simulink model "power_2rectifiers"  (Simulink 6.0)
settings: Solver=ode23tb  SolverMode=SingleTasking  StartTime=0.0  StopTime=0.1  RelTol=1e-3
libraries: powerlib x25
settings Model: Creator=sybille  LastModifiedBy=batserve  ExtModeTrigMode=oneshot  ExtModeArmWhenConnect=off  ExtModeAutoUpdateStatusClock=off
settings DataIOCC: LimitDataPoints=off  SignalLoggingName=sigsOut
settings OptimizationCC: BlockReduction=off  BooleanDataType=off
settings DebuggingCC: CheckExecutionContextPreStartOutputMsg=on  CheckExecutionContextRuntimeOutputMsg=on  SolverPrmCheckMsg=none
settings HardwareCC: TargetUnknown=on

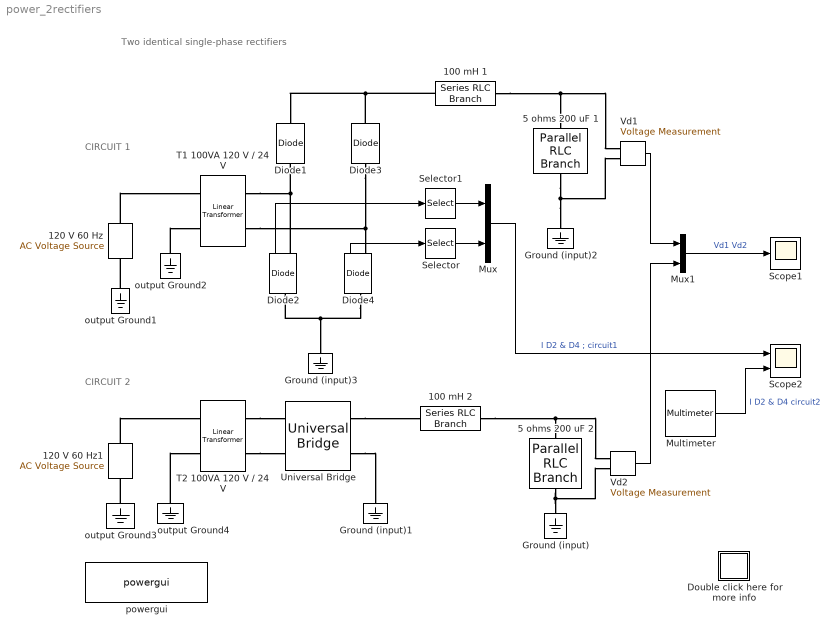
== system power_2rectifiers ==
  note: CIRCUIT 1
  note: CIRCUIT 2
  note: Two identical single-phase rectifiers
  100 mH 1 : powerlib/Elements/Series RLC Branch  PhysicalDomain=powersysdomain  SubClassName=unknown  LeftPortType=p1  RightPortType=p1  LConnTagsString=__new0  RConnTagsString=__new0  Resistance=0  Inductance=100e-03  Capacitance=inf  Measurements=None
  100 mH 2 : powerlib/Elements/Series RLC Branch  PhysicalDomain=powersysdomain  SubClassName=unknown  LeftPortType=p1  RightPortType=p1  LConnTagsString=__new0  RConnTagsString=__new0  Resistance=0  Inductance=100e-03  Capacitance=inf  Measurements=None
  120 V 60 Hz : powerlib/Electrical Sources/AC Voltage Source  Description=source block  Orientation=up  Amplitude=120*sqrt(2)  Phase=0  Frequency=60  SampleTime=0  Measurements=None
      settings: AttributesFormatString=\n
  120 V 60 Hz1 : powerlib/Electrical Sources/AC Voltage Source  Description=source block  Orientation=up  Amplitude=120*sqrt(2)  Phase=0  Frequency=60  SampleTime=0  Measurements=None
      settings: AttributesFormatString=\n
  5 ohms 200 uF 1 : powerlib/Elements/Parallel RLC Branch  Orientation=down  PhysicalDomain=powersysdomain  SubClassName=unknown  LeftPortType=p1  RightPortType=p1  LConnTagsString=a  RConnTagsString=__new0  Resistance=5  Inductance=inf  Capacitance=200e-06  Measurements=None
  5 ohms 200 uF 2 : powerlib/Elements/Parallel RLC Branch  Orientation=down  PhysicalDomain=powersysdomain  SubClassName=unknown  LeftPortType=p1  RightPortType=p1  LConnTagsString=a  RConnTagsString=__new0  Resistance=5  Inductance=inf  Capacitance=200e-06  Measurements=None
  Diode1 : powerlib/Power Electronics/Diode  Orientation=up  Ron=0.01  Lon=0  Vf=0.8  IC=0  Rs=250  Cs=0.1e-6  Measurements=off
  Diode2 : powerlib/Power Electronics/Diode  Orientation=up  Ron=0.01  Lon=0  Vf=0.8  IC=0  Rs=250  Cs=0.1e-6  Measurements=on
  Diode3 : powerlib/Power Electronics/Diode  Orientation=up  Ron=0.01  Lon=0  Vf=0.8  IC=0  Rs=250  Cs=0.1e-6  Measurements=off
  Diode4 : powerlib/Power Electronics/Diode  Orientation=up  Ron=0.01  Lon=0  Vf=0.8  IC=0  Rs=250  Cs=0.1e-6  Measurements=on
  Double click here for more info : Subsystem
      mask Display: disp('?')
  Ground (input){,1..3} (4 alike) : powerlib/Elements/Ground  Orientation=down  PhysicalDomain=powersysdomain  SubClassName=unknown  LeftPortType=p1  RightPortType=p1  LConnTagsString=a
  Multimeter : powerlib/Measurements/Multimeter  Tag=PoWeRsYsTeMmEaSuReMeNt  PhasorSimulation=off  OutputType=Magnitude  sel=[2 4]  L=4  Gain=[1 1]  yselected={'Isw2: Universal Bridge','Isw4: Universal Bridge'};  PSBOutputType=1  PSBequivalent=0  AxesSetting=[0,0.1,-100,100]  Display=0  SavedBlockNames=-11
      settings: AttributesFormatString=\n
  Mux : Mux  Inputs=2
  Mux1 : Mux  Inputs=2
  Scope1 : Scope
      settings: TimeRange=0.1  YMin=0  YMax=20  SaveName=V2X  DataFormat=Array  SampleInput=on  SampleTime=10e-6
  Scope2 : Scope  NumInputPorts=2
      settings: TimeRange=0.1  YMin=0~0  YMax=4~4  SaveName=V2X  DataFormat=Array  SampleInput=on  SampleTime=10e-6
  Selector : Selector  InputPortWidth=2
  Selector1 : Selector  InputPortWidth=2
  T1 100VA 120 V / 24 V : powerlib/Elements/Linear Transformer  PhysicalDomain=powersysdomain  SubClassName=unknown  LeftPortType=p1  RightPortType=p1  LConnTagsString=a|b  RConnTagsString=A|B  NominalPower=[100 60]  winding1=[120 0.03 0.02]  winding2=[24 0.03 0.02]  ThreeWindings=off  winding3=[24 0.03 0.02]  RmLm=[25 25]  Measurements=None
  T2 100VA 120 V / 24 V : powerlib/Elements/Linear Transformer  PhysicalDomain=powersysdomain  SubClassName=unknown  LeftPortType=p1  RightPortType=p1  LConnTagsString=a|b  RConnTagsString=A|B  NominalPower=[100 60]  winding1=[120 0.03 0.02]  winding2=[24 0.03 0.02]  ThreeWindings=off  winding3=[24 0.03 0.02]  RmLm=[25 25]  Measurements=None
  Universal Bridge : powerlib/Power Electronics/Universal Bridge  Arms=2  SnubberResistance=250  SnubberCapacitance=0.1e-6  Device=Diodes  Ron=0.01  Lon=0  ForwardVoltages="[  0.8  0.8  ]"  ForwardVoltage=0.8  GTOparameters=[ 10e-6 , 20e-6 ]  IGBTparameters=[ 1e-6 , 2e-6 ]  Measurements=Device currents
  Vd1 : powerlib/Measurements/Voltage Measurement  Tag=PoWeRsYsTeMmEaSuReMeNt  PhasorSimulation=off  OutputType=Magnitude  PSBequivalent=0
  Vd2 : powerlib/Measurements/Voltage Measurement  Tag=PoWeRsYsTeMmEaSuReMeNt  PhasorSimulation=off  OutputType=Magnitude  PSBequivalent=0
  output Ground{1..4} (4 alike) : powerlib/Elements/Ground  Orientation=down  PhysicalDomain=powersysdomain  SubClassName=unknown  LeftPortType=p1  RightPortType=p1  LConnTagsString=a
  powergui : powerlib/powergui  Priority=2  Frange=[0:2:500]  Ylog=off  Xlog=on  save=off  variable=ZData  ZoomFFT=on  StartTime=0.0  cycles=1  DisplayStyle=off  fundamental=60  FreqAxis=off  MaxFrequency=1000  frequencyindice=1  frequencyindicesteady=1  RmsSteady=1  display=off  Ts=50e-6  methode=off  frequency=60  echomessages=on
  wires:
  Selector1/1 -> Mux/1
  Selector/1 -> Mux/2
  Mux/1 -> Scope2/1  "I D2 & D4 ; circuit1"
  Mux1/1 -> Scope1/1  "Vd1 Vd2"
  Diode4/1 -> Selector/1
  Diode2/1 -> Selector1/1
  Multimeter/1 -> Scope2/2  "I D2 & D4 circuit2"
  Vd1/1 -> Mux1/1
  Vd2/1 -> Mux1/2
  connections:
  120 V 60 Hz/RConn1 -- T1 100VA 120 V / 24 V/LConn1
  output Ground1/LConn1 -- 120 V 60 Hz/LConn1
  output Ground2/LConn1 -- T1 100VA 120 V / 24 V/LConn2
  120 V 60 Hz1/RConn1 -- T2 100VA 120 V / 24 V/LConn1
  output Ground3/LConn1 -- 120 V 60 Hz1/LConn1
  output Ground4/LConn1 -- T2 100VA 120 V / 24 V/LConn2
  T2 100VA 120 V / 24 V/RConn2 -- Universal Bridge/LConn2
  T2 100VA 120 V / 24 V/RConn1 -- Universal Bridge/LConn1
  Ground (input)/LConn1 -- 5 ohms 200 uF 2/RConn1 -- Vd2/LConn2
  Universal Bridge/RConn1 -- 100 mH 2/LConn1
  100 mH 2/RConn1 -- 5 ohms 200 uF 2/LConn1 -- Vd2/LConn1
  100 mH 1/RConn1 -- 5 ohms 200 uF 1/LConn1 -- Vd1/LConn1
  5 ohms 200 uF 1/RConn1 -- Vd1/LConn2 -- Ground (input)2/LConn1
  Diode3/LConn1 -- Diode4/RConn1 -- T1 100VA 120 V / 24 V/RConn2
  Diode2/RConn1 -- Diode1/LConn1 -- T1 100VA 120 V / 24 V/RConn1
  100 mH 1/LConn1 -- Diode1/RConn1 -- Diode3/RConn1
  Diode4/LConn1 -- Diode2/LConn1 -- Ground (input)3/LConn1
  Universal Bridge/RConn2 -- Ground (input)1/LConn1

== system power_2rectifiers/Double click here for more info ==
  note: This demonstration illustrates use of the Universal Bridge, Multimeter,
      | and Discrete System blocks
  note: Demonstration
  note: Circuit Description
  note: This system contains two identical circuits showing the operation of a single phase rectifier.
      |
      | The rectifiers are fed by a 120 V/ 24 V linear transformer. The rectified voltage is filtered by a
      | 100 mH / 200 uF filter and applied to a 5 ohm resistive load. The load voltages are measured
      | by two Voltage Measurement blocks Vd1 and Vd2.
      |
      | The top circuit (circuit 1) uses four individual diodes connected in a bridge configuration.
      | The currents of diodes 2 and 4 are obtained at the measurement 'm' output of the diode blocks
      | and sent to input 1 of Scope 2 through Selector and Multiplex blocks.
      |
      | The bottom circuit (circuit 2) is functiunally identical to circuit 1, but the circuit assembly is
      | considerably simplified by the use of the Universal Bridge.
  note: Open the Universal Bridge dialog box and notice that in order to obtain a four-diode bridge configuration,
      | the Power electronic devices field has been set to 'Diodes' and  that the number of arms has been set to 2.
      | Also, observe that the Measurements field has been set to 'Device currents', thus allowing
      | measurement of  diode currents through the Multimeter block.
      |
      | Now, double click on the Multimeter block. The four diode currents are listed in the left column.
      | Notice that only currents in diodes 2 and 4 have been selected and transferred in the right column.
      | The number of available signals at the multimeter output (2) is displayed on the block icon.
      |
      | Open the two scopes and start the simulation. Compare the two load voltages Vd1 and Vd2 which are
      | superimposed on Scope1. Also, compare on Scope2 the currents flowing in diodes 2 and 4  for
      | circuit 1 and circuit 2.
      |
      | Notice that the circuit has been discretized by means of the Powergui  block. The sample time (50e-6 s)
      | appears on the block icon.
      |
      | Now, open the Powergui block and  deselect  'Discretize electrical model'.  The continuous ode23tb solver specified
      | in the Simulation parameters will now be used.  Restart the simulation and compare the continuous simulation results
      |  with the previous simulation results obtained with a discretized system.
  note: G. Sybille (Hydro-Quebec)
